simulink model "cartpole"  (R2018a)
settings: Solver=FixedStepAuto  StartTime=0.0  StopTime=10.0  FixedStep=0.02  RelTol=1e-3
values from neighbouring files (symbols this model uses):
  f_threshold = [-30 30]    [cartpole_params.mat]
  g = 9.8    [cartpole_params.mat]
  l_cg = 0.5    [cartpole_params.mat]
  m_cart = 1    [cartpole_params.mat]
  m_pendulum = 0.1    [cartpole_params.mat]
  theta_o = 0    [cartpole_params.mat]
  theta_threshold_radians = 0.209439510239    [cartpole_params.mat]
  thetadot_o = 0    [cartpole_params.mat]
  x_o = 0    [cartpole_params.mat]
  x_threshold = 2.4    [cartpole_params.mat]
  xdot_o = 0    [cartpole_params.mat]
settings Model: TunableVars=f_threshold,g,l_cg,m_cart,m_pendulum,theta_o,theta_threshold_radians,thetadot_o,x_o,x_threshold,xdot_o  TunableVarsStorageClass=Auto,Auto,Auto,Auto,Auto,Auto,Auto,Auto,Auto,Auto,Auto  TunableVarsTypeQualifier=,,,,,,,,,,  OrderedModelArguments=off  Creator=hjzsj  LastModifiedBy=JieLi
settings DataIOCC: ReturnWorkspaceOutputs=on
settings OptimizationCC: DefaultParameterBehavior=Inlined  UseDivisionForNetSlopeComputation=on  UseFloatMulNetSlope=on  PassReuseOutputArgsAs=Individual arguments  NoFixptDivByZeroProtection=on  EfficientFloat2IntCast=on  LifeSpan=1  OptimizeBlockOrder=speed  DifferentSizesBufferReuse=on
settings DebuggingCC: ParameterTunabilityLossMsg=error
settings HardwareCC: ProdLongLongMode=on
settings SFSimCC: SimUseLocalCustomCode=on  MATLABDynamicMemAlloc=off
settings RTWCC: SystemTargetFile=ert.tlc  GenCodeOnly=on  TemplateMakefile=ert_default_tmf  RTWUseLocalCustomCode=on  TargetLang=C++
settings CodeAppCC: ForceParamTrailComments=on  IgnoreCustomStorageClasses=off  OperatorAnnotations=on  SimulinkDataObjDesc=on  SFDataObjDesc=on  CustomSymbolStrGlobalVar=rt$N$M  CustomSymbolStrType=$N$M  CustomSymbolStrFcn=$N$M$F  CustomSymbolStrMacro=$N$M  InsertBlockDesc=on
settings ERTTargetCC: TargetLangStandard=C++03 (ISO)  GenerateSampleERTMain=on  CombineSignalStateStructs=on  SupportAbsoluteTime=off  MultiInstanceERTCode=on  CodeInterfacePackaging=C++ class  SupportComplex=off  SupportContinuousTime=on  InlinedParameterPlacement=NonHierarchical  RootIOFormat=Structure reference  ERTCustomFileTemplate=example_file_process.tlc  ERTFilePackagingFormat=CompactWithDataFile

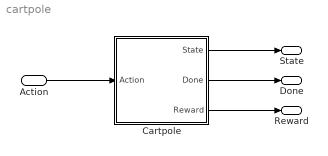
== system cartpole ==
  Action : Inport
  Cartpole : Subsystem  mask(Inverted pendulum on cart){Mcart=m_cart, m=m_pendulum, l=l_cg, g=g, x_threshold=x_threshold, theta_threshold_radians=theta_threshold_radians}
      mask prompts: Mcart "Mass of cart (kg):"; m "Mass of pendulum (kg):"; l "Distance to pendulum center of mass(m):"; g "Acceleration of gravity (m/s^2):"; x_threshold "Reset threshold of x (m)"; theta_threshold_radians "Reset threshold of theta"
      mask help: Unmask and double-click to see dynamics
      mask Help: Nonlinear dynamics of inverted pendulum on cart.
  State : Outport  VectorParamsAs1DForOutWhenUnconnected=on
  Done : Outport  Port=2  VectorParamsAs1DForOutWhenUnconnected=on
  Reward : Outport  Port=3  VectorParamsAs1DForOutWhenUnconnected=on
  wires:
  Cartpole/1(State) -> State/1
  Cartpole/2(Done) -> Done/1
  Cartpole/3(Reward) -> Reward/1
  Action/1 -> Cartpole/1(Action)

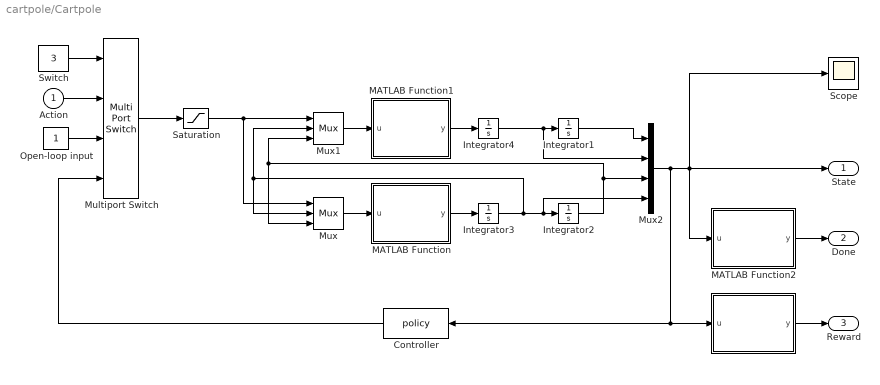
== system cartpole/Cartpole ==
  Action : Inport
  " " : MATLAB Function  TreatAsAtomicUnit=on
  Controller : S-Function  FunctionName=policy  SFunctionDeploymentMode=off  EnableBusSupport=off
  Integrator1 : Integrator  InitialCondition=x_o
  Integrator2 : Integrator  InitialCondition=theta_o
  Integrator3 : Integrator  InitialCondition=thetadot_o
  Integrator4 : Integrator  InitialCondition=xdot_o
  MATLAB Function : MATLAB Function  TreatAsAtomicUnit=on
  MATLAB Function1 : MATLAB Function  TreatAsAtomicUnit=on
  MATLAB Function2 : MATLAB Function  TreatAsAtomicUnit=on
  Multiport Switch : MultiPortSwitch
  Mux : Mux  Inputs=3
  Mux1 : Mux  Inputs=3
  Mux2 : Mux
  Open-loop input : Constant
  Saturation : Saturate  UpperLimit=f_threshold(2)  LowerLimit=f_threshold(1)
  Scope : Scope
  Switch : Constant  Value=3
  State : Outport  VectorParamsAs1DForOutWhenUnconnected=on
  Done : Outport  Port=2  VectorParamsAs1DForOutWhenUnconnected=on
  Reward : Outport  Port=3  VectorParamsAs1DForOutWhenUnconnected=on
  wires:
  MATLAB Function/1(y) -> Integrator3/1
  Mux/1 -> MATLAB Function/1(u)
  Mux1/1 -> MATLAB Function1/1(u)
  MATLAB Function1/1(y) -> Integrator4/1
  Integrator4/1 -> Mux2/2, Integrator1/1
  Action/1 -> Multiport Switch/2
  Integrator3/1 -> Mux2/4, Integrator2/1, Mux1/2, Mux/2
  Integrator2/1 -> Mux1/3, Mux/3, Mux2/3
  Integrator1/1 -> Mux2/1
  MATLAB Function2/1(y) -> Done/1
  " "/1(y) -> Reward/1
  Mux2/1 -> Controller/1, " "/1(u), Scope/1, MATLAB Function2/1(u), State/1
  Saturation/1 -> Mux1/1, Mux/1
  Switch/1 -> Multiport Switch/1
  Open-loop input/1 -> Multiport Switch/3
  Multiport Switch/1 -> Saturation/1
  Controller/1 -> Multiport Switch/4

== matlab function cartpole/Cartpole/MATLAB Function1 ==
  data: u input size=3; y output; Mcart parameter; m parameter; l parameter; g parameter
function y = fcn(u, Mcart, m, l, g)
y = (u(1)/m - g*sin(u(3))*cos(u(3)) + l*power(u(2),2)*sin(u(3)))/(Mcart/m + power(sin(u(3)),2));

== matlab function cartpole/Cartpole/MATLAB Function ==
  data: u input size=3; y output; Mcart parameter; m parameter; l parameter; g parameter
function y = fcn(u, Mcart, m, l, g)
y = (-u(1)*cos(u(3))/m + (Mcart+m)*g*sin(u(3))/m - l*power(u(2),2)*sin(u(3))*cos(u(3)))/(l*(Mcart/m + power(sin(u(3)),2)));

== matlab function cartpole/Cartpole/MATLAB Function2 ==
  data: u input size=4; y output; theta_threshold_radians parameter; x_threshold parameter
function y = fcn(u, theta_threshold_radians, x_threshold)
done = (abs(u(1)) > x_threshold)||(abs(u(3)) > theta_threshold_radians)
y = done

== matlab function cartpole/Cartpole/  ==
  data: u input size=4; y output; theta_threshold_radians parameter; x_threshold parameter
function y = fcn(u, theta_threshold_radians, x_threshold)
done = (abs(u(1)) > x_threshold)||(abs(u(3)) > theta_threshold_radians)
y = 1 - double(done)
